simulink model "Fourier_Series_Square_Wave"  (Simulink 10.1)
settings: Solver=VariableStepAuto  StartTime=0.0  StopTime=100.0  RelTol=1e-3
settings Model: Creator=Micheal  LastModifiedBy=Micheal
settings DataIOCC: SaveFormat=Dataset  ReturnWorkspaceOutputs=on
settings OptimizationCC: LifeSpan=auto
settings DebuggingCC: UnderspecifiedInitializationDetection=Simplified  MergeDetectMultiDrivingBlocksExec=error  SFUnexpectedBacktrackingDiag=error  SFNoUnconditionalDefaultTransitionDiag=error  SFExecutionAtInitializationDiag=warning  ArithmeticOperatorsInVariantConditions=error
settings HardwareCC: ProdBitPerPointer=64  ProdBitPerSizeT=64  ProdBitPerPtrDiffT=64  ProdLargestAtomicFloat=Float  ProdIntDivRoundTo=Zero  ProdEndianess=LittleEndian  ProdWordSize=64  ProdHWDeviceType=Intel->x86-64 (Windows64)
settings ModelReferenceCC: PropagateSignalLabelsOutOfModel=on
settings SFSimCC: SimUseLocalCustomCode=on  CustomCodeUndefinedFunction=FilterOut
settings RTWCC: RTWUseLocalCustomCode=on
settings CodeAppCC: StateflowObjectComments=off
settings GRTTargetCC: TargetLangStandard=C99 (ISO)  CombineOutputUpdateFcns=on  GRTInterface=off
settings ConfigComp: CovMetricSettings=dwe  CovHtmlReporting=off  CovSaveCumulativeToWorkspaceVar=off  CovSaveSingleToWorkspaceVar=off  CovExternalEMLEnable=on

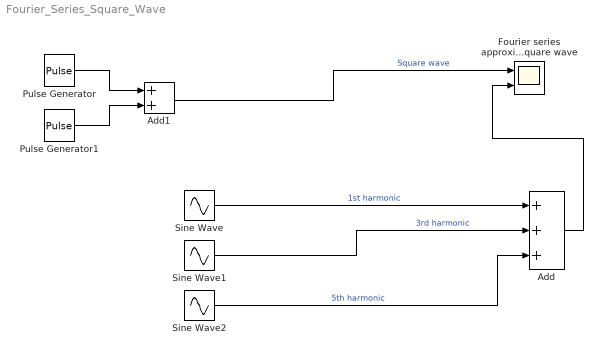
== system Fourier_Series_Square_Wave ==
  Add : Sum  Inputs=+++
  Add1 : Sum
  Fourier series approximation of square wave : Scope  NumInputPorts=2
  Pulse Generator : DiscretePulseGenerator  PulseType=Time based  Period=10  PulseWidth=50
  Pulse Generator1 : DiscretePulseGenerator  PulseType=Time based  Amplitude=-1  Period=10  PulseWidth=50  PhaseDelay=5
  Sine Wave : Sin  Amplitude=4/pi  Frequency=2*pi/10  SampleTime=0
  Sine Wave1 : Sin  Amplitude=4/(3*pi)  Frequency=6*pi/(10)  SampleTime=0
  Sine Wave2 : Sin  Amplitude=4/(5*pi)  Frequency=10*pi/10  SampleTime=0
  wires:
  Pulse Generator/1 -> Add1/1
  Sine Wave/1 -> Add/1  "1st harmonic"
  Sine Wave1/1 -> Add/2  "3rd harmonic"
  Add/1 -> Fourier series approximation of square wave/2
  Sine Wave2/1 -> Add/3  "5th harmonic"
  Pulse Generator1/1 -> Add1/2
  Add1/1 -> Fourier series approximation of square wave/1  "Square wave"
